simulink model "sim_model"  (Simulink 9.0)
settings: Solver=ode45  StartTime=0.0  StopTime=10  RelTol=1e-3  EnableMultiTasking=on
libraries: simulink x3
settings Model: Creator=DYBLENKO  LastModifiedBy=userus
settings DataIOCC: LimitDataPoints=on  SignalLoggingSaveFormat=ModelDataLogs  SignalLoggingName=sigsOut
settings OptimizationCC: ExpressionDepthLimit=2147483647  InitFltsAndDblsToZero=on
settings DebuggingCC: SaveWithParameterizedLinksMsg=none  SignalResolutionControl=TryResolveAllWithWarning  MultiTaskDSMMsg=warning  MultiTaskCondExecSysMsg=none  FcnCallInpInsideContextMsg=warning  StateNameClashWarn=warning  StrictBusMsg=None
settings HardwareCC: TargetUnknown=on
settings GRTTargetCC: CombineOutputUpdateFcns=off  GRTInterface=on

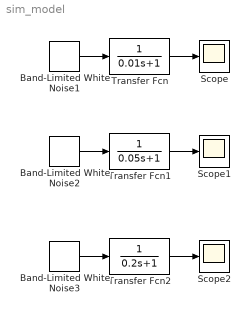
== system sim_model ==
  Band-Limited White Noise1 : simulink/Sources/Band-Limited White Noise  Cov=[1*2*0.01]  Ts=.01/100  seed=[23341]
  Band-Limited White Noise2 : simulink/Sources/Band-Limited White Noise  Cov=[1*2*0.05]  Ts=.01/100  seed=[23341]
  Band-Limited White Noise3 : simulink/Sources/Band-Limited White Noise  Cov=[1*2*.2]  Ts=.01/100  seed=[23341]
  Scope : Scope
  Scope1 : Scope
  Scope2 : Scope
  Transfer Fcn : TransferFcn  Denominator=[0.01 1]
  Transfer Fcn1 : TransferFcn  Denominator=[0.05 1]
  Transfer Fcn2 : TransferFcn  Denominator=[0.2 1]
  wires:
  Transfer Fcn/1 -> Scope/1
  Band-Limited White Noise1/1 -> Transfer Fcn/1
  Transfer Fcn1/1 -> Scope1/1
  Band-Limited White Noise2/1 -> Transfer Fcn1/1
  Transfer Fcn2/1 -> Scope2/1
  Band-Limited White Noise3/1 -> Transfer Fcn2/1
